simulink model "feedback_lin_EKF"  (R2023b)
settings: Solver=VariableStepAuto  StartTime=0.0  StopTime=2  RelTol=1e-3
values from neighbouring files (symbols this model uses):
  A_ob = A - L*C    [main_feedback_lin.m]
  B_ob = [ B - L*D, L]    [main_feedback_lin.m]
  C_ob = eye(n)    [main_feedback_lin.m]
  D_ob = zeros(n, m+p)    [main_feedback_lin.m]
  m = 1    [main_feedback_lin.m]
undefined symbols (not defined in the file or in its folder): k_aero, k_mag, Lc, Rtot, x1_eq0, x2_eq0, y0
libraries: simulink x3
settings Model: Creator=lollo  LastModifiedBy=lollo

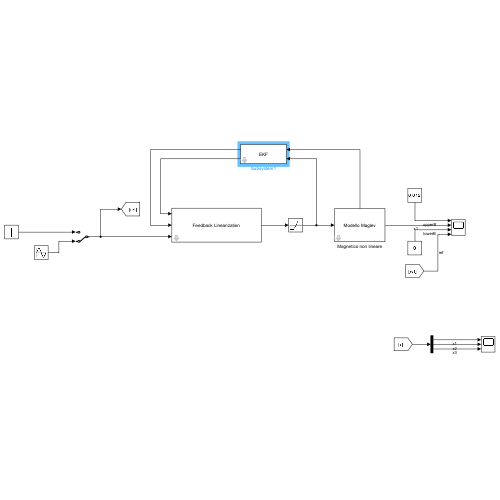
[thumbnail: Simulink's stored preview of the top-level diagram]
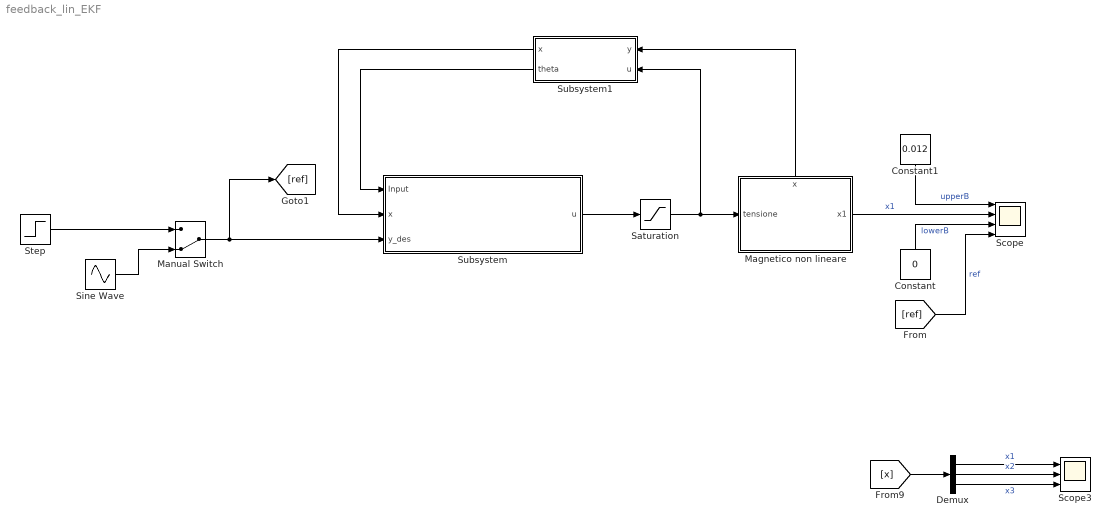
== system feedback_lin_EKF ==
  Constant : Constant  Value=0
  Constant1 : Constant  Value=0.012
  Demux : Demux  Outputs=3
  Magnetico non lineare : Subsystem  mask{dist=on, obs=on, k_aero=k_aero, k_mag=k_mag, m=m, y0=y0, Rtot=Rtot, Lc=Lc}
      mask prompts: dist "Aggiungere Disturbi"; obs "Observer invece di misura"
      settings: PortSchema="{\"entries\":[{\"content\":{\"sides\":[{\"content\":{\"connectorIds\":[\"In1\"]},\"type\":\"ConnectorPlacement.EquallySpacedRectSide\",\"uuid\":\"4c2628b7-19c4-4753-accd-078547eff280\"},{\"content\":{\"connectorIds\":[\"Out1\"],\"side\":\"RIGHT\"},\"type\":\"ConnectorPlacement.EquallySpacedRectSide\",\"uuid\":\"46f8a782-99b4-4db5-ac9e-879226864e1a\"},{\"content\":{\"connectorIds\":[\"Out2\"],\"side\":\"TOP\"},\"type\":\"ConnectorPlacement.EquallySpacedRectSide\",\"uuid\":\"e9ea6a3a-0b10-4f27-be26-5b91ce6de957\"}]},\"type\":\"ConnectorPlacement.EquallySpacedConnector\",\"uuid\":\"8380a659-82e1-48e4-be7e-4b84feeb9f50\"}],\"packageUris\":[\"http://schema.mathworks.com/mf0/Connector/R2020b\"],\"version\":\"1.0\"}"
      mask DialogControl DescGroupVar Prompt: MAGLEV
      mask DialogControl Maglev Prompt: Possibilità di aggiungere disturbi alla misura o di considerare gli observer (solo ridotto alla velocità). Inoltre possibilità di modificare i parametri del modello per testare robustezza
      mask DialogControl Disturbi Prompt: Disturbi
      mask DialogControl Parametri Prompt: Parametri Modello
      mask Display: disp('Modello Maglev')
  Manual Switch : ManualSwitch  CurrentSetting=0
  Saturation : Saturate  UpperLimit=23  LowerLimit=0
  Scope : Scope  NumInputPorts=4
  Scope3 : Scope  NumInputPorts=3
  Sine Wave : Sin  Amplitude=0.001  Bias=0.004  Frequency=10  SampleTime=0
  Step : Step  Time=0  After=0.008  SampleTime=0
  Subsystem : Subsystem  mask{tau=0.003, p1=-100, p2=-60, p3=-70}
      mask DialogControl DescGroupVar Prompt: Feedback Linearization
      mask DialogControl DescTextVar Prompt: Tau corrisponde al tempo caratteristico del filtro per il calcolo delle derivate. k1, k2, k3 sono i poli della feedback linearization dei rispettivi stati
      mask Display: disp('Feedback Linearization')
  Subsystem1 : Subsystem
      mask Display: disp('EKF')
  wires:
  Magnetico non lineare/1(x1) -> Scope/2  "x1"
  Manual Switch/1 -> [ref], Subsystem/3(y_des)
  Subsystem/1(u) -> Saturation/1
  Saturation/1 -> Subsystem1/2(u), Magnetico non lineare/1(tensione)
  Constant/1 -> Scope/3  "lowerB"
  Constant1/1 -> Scope/1  "upperB"
  [x] -> Demux/1
  Demux/2 -> Scope3/2  "x2"
  Demux/3 -> Scope3/3  "x3"
  Demux/1 -> Scope3/1  "x1"
  [ref] -> Scope/4  "ref"
  Step/1 -> Manual Switch/1
  Sine Wave/1 -> Manual Switch/2
  Magnetico non lineare/2(x) -> Subsystem1/1(y)
  Subsystem1/1(x) -> Subsystem/2(x)
  Subsystem1/2(theta) -> Subsystem/1(Input)

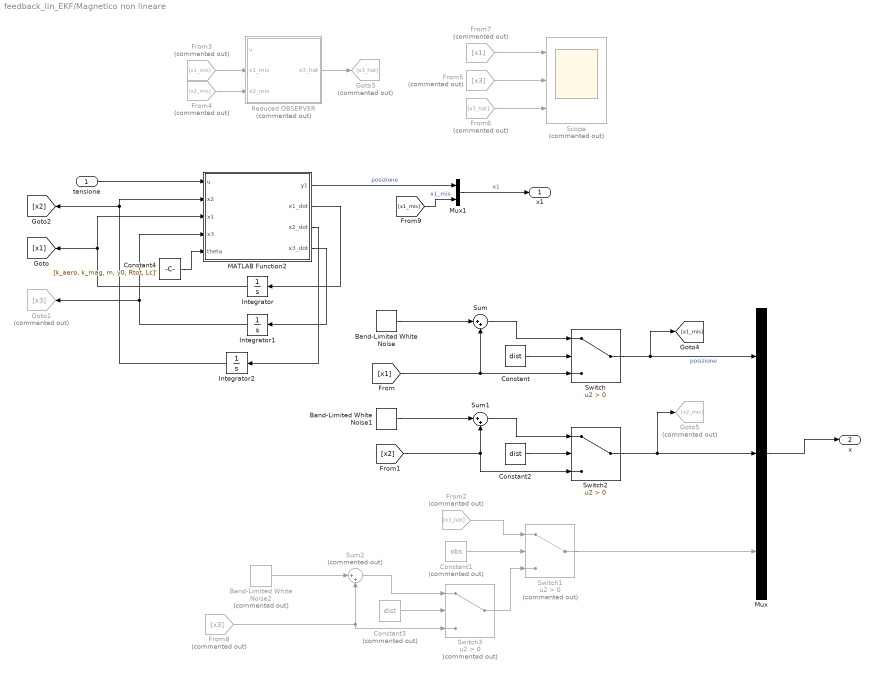
== system feedback_lin_EKF/Magnetico non lineare ==
  tensione : Inport
  Band-Limited White Noise : simulink/Sources/Band-Limited White Noise  Cov=[8.9934e-11*0.002]  Ts=0.002  seed=[23341]
  Band-Limited White Noise1 : simulink/Sources/Band-Limited White Noise  Cov=[8.9934e-11*0.002]  Ts=0.002  seed=[23341]
  Band-Limited White Noise2 : simulink/Sources/Band-Limited White Noise  Commented=on  Cov=[8.9934e-11*0.002]  Ts=0.002  seed=[23341]
  Constant : Constant  Value=dist
  Constant1 : Constant  Commented=on  Value=obs
  Constant2 : Constant  Value=dist
  Constant3 : Constant  Commented=on  Value=dist
  Constant4 : Constant  Value=[k_aero, k_mag, m, y0, Rtot, Lc]'
  From2 : From  Commented=on  GotoTag=x3_hat
  From3 : From  Commented=on  GotoTag=x1_mis
  From4 : From  Commented=on  GotoTag=x2_mis
  From5 : From  Commented=on  GotoTag=x3
  From6 : From  Commented=on  GotoTag=x3_hat
  From7 : From  Commented=on  GotoTag=x1
  From8 : From  Commented=on  GotoTag=x3
  Goto1 : Goto  Commented=on  GotoTag=x3
  Goto3 : Goto  Commented=on  GotoTag=x3_hat
  Goto5 : Goto  Commented=on  GotoTag=x2_mis
  Integrator : Integrator
  Integrator1 : Integrator
  Integrator2 : Integrator
  MATLAB Function2 : MATLAB Function  TreatAsAtomicUnit=on
  Mux : Mux  Inputs=3
  Mux1 : Mux  Inputs=2
  Reduced OBSERVER : Subsystem  Commented=on
  Scope : Scope  Commented=on  NumInputPorts=3
  Sum : Sum  Inputs=|++
  Sum1 : Sum  Inputs=|++
  Sum2 : Sum  Commented=on  Inputs=|++
  Switch : Switch  Criteria=u2 > Threshold  SaturateOnIntegerOverflow=off  InputSameDT=off
  Switch1 : Switch  Commented=on  Criteria=u2 > Threshold  SaturateOnIntegerOverflow=off  InputSameDT=off
  Switch2 : Switch  Criteria=u2 > Threshold  SaturateOnIntegerOverflow=off  InputSameDT=off
  Switch3 : Switch  Commented=on  Criteria=u2 > Threshold  SaturateOnIntegerOverflow=off  InputSameDT=off
  x1 : Outport
  x : Outport  Port=2
  wires:
  tensione/1 -> MATLAB Function2/1(u)
  Switch/1 -> [x1_mis], Mux/1  "posizione"
  MATLAB Function2/2(x1_dot) -> Integrator/1
  Integrator/1 -> MATLAB Function2/3(x1), [x1]
  MATLAB Function2/4(x3_dot) -> Integrator1/1
  Integrator1/1 -> Goto1/1, MATLAB Function2/4(x3)
  [x1] -> Sum/2, Switch/3
  From2/1 -> Switch1/1
  Mux/1 -> x/1
  MATLAB Function2/3(x2_dot) -> Integrator2/1
  From3/1 -> Reduced OBSERVER/2(x1_mis)
  From4/1 -> Reduced OBSERVER/3(x2_mis)
  Reduced OBSERVER/1(x3_hat) -> Goto3/1
  From6/1 -> Scope/3
  From5/1 -> Scope/2
  Integrator2/1 -> [x2], MATLAB Function2/2(x2)
  From7/1 -> Scope/1
  Constant/1 -> Switch/2
  Band-Limited White Noise/1 -> Sum/1
  Sum/1 -> Switch/1
  Constant1/1 -> Switch1/2
  Switch1/1 -> Mux/3
  Constant2/1 -> Switch2/2
  Switch2/1 -> Goto5/1, Mux/2
  Band-Limited White Noise1/1 -> Sum1/1
  Sum1/1 -> Switch2/1
  [x2] -> Sum1/2, Switch2/3
  Constant3/1 -> Switch3/2
  Switch3/1 -> Switch1/3
  Band-Limited White Noise2/1 -> Sum2/1
  Sum2/1 -> Switch3/1
  From8/1 -> Sum2/2, Switch3/3
  [x1_mis] -> Mux1/2  "x1_mis"
  MATLAB Function2/1(y1) -> Mux1/1  "posizione"
  Mux1/1 -> x1/1  "x1"
  Constant4/1 -> MATLAB Function2/5(theta)

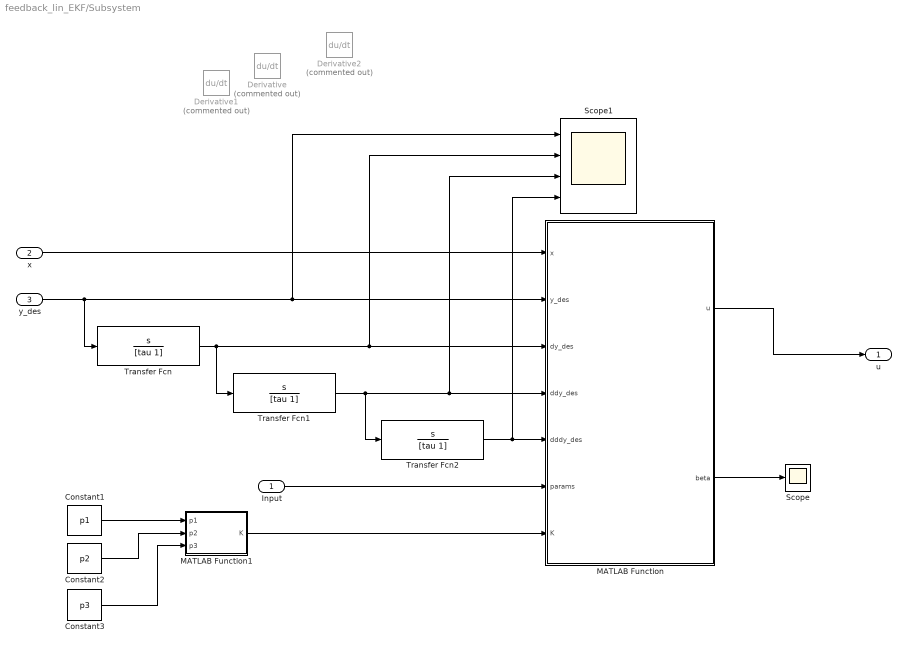
== system feedback_lin_EKF/Subsystem ==
  Input : Inport
  x : Inport  Port=2
  y_des : Inport  Port=3
  Constant1 : Constant  Value=p1
  Constant2 : Constant  Value=p2
  Constant3 : Constant  Value=p3
  Derivative : Derivative  Commented=on
  Derivative1 : Derivative  Commented=on
  Derivative2 : Derivative  Commented=on
  MATLAB Function : MATLAB Function  TreatAsAtomicUnit=on
  MATLAB Function1 : MATLAB Function  TreatAsAtomicUnit=on
  Scope : Scope
  Scope1 : Scope  NumInputPorts=4
  Transfer Fcn : TransferFcn  Numerator=[1 0]  Denominator=[tau 1]
  Transfer Fcn1 : TransferFcn  Numerator=[1 0]  Denominator=[tau 1]
  Transfer Fcn2 : TransferFcn  Numerator=[1 0]  Denominator=[tau 1]
  u : Outport
  wires:
  y_des/1 -> Transfer Fcn/1, MATLAB Function/2(y_des), Scope1/1
  x/1 -> MATLAB Function/1(x)
  MATLAB Function/1(u) -> u/1
  Transfer Fcn/1 -> MATLAB Function/3(dy_des), Scope1/2, Transfer Fcn1/1
  Input/1 -> MATLAB Function/6(params)
  Transfer Fcn1/1 -> Transfer Fcn2/1, Scope1/3, MATLAB Function/4(ddy_des)
  MATLAB Function/2(beta) -> Scope/1
  Transfer Fcn2/1 -> Scope1/4, MATLAB Function/5(dddy_des)
  MATLAB Function1/1(K) -> MATLAB Function/7(K)
  Constant3/1 -> MATLAB Function1/3(p3)
  Constant2/1 -> MATLAB Function1/2(p2)
  Constant1/1 -> MATLAB Function1/1(p1)

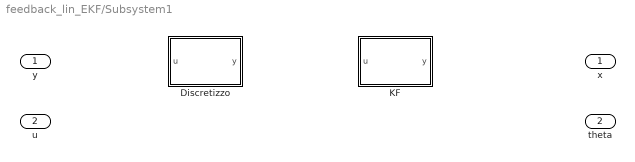
== system feedback_lin_EKF/Subsystem1 ==
  y : Inport
  u : Inport  Port=2
  Discretizzo : MATLAB Function  TreatAsAtomicUnit=on
  KF : MATLAB Function  TreatAsAtomicUnit=on
  x : Outport
  theta : Outport  Port=2

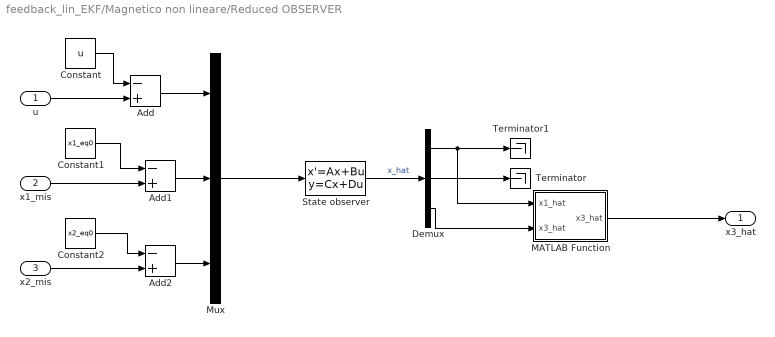
== system feedback_lin_EKF/Magnetico non lineare/Reduced OBSERVER ==
  u : Inport
  x1_mis : Inport  Port=2
  x2_mis : Inport  Port=3
  Add : Sum  Inputs=-+
  Add1 : Sum  Inputs=-+
  Add2 : Sum  Inputs=-+
  Constant : Constant  Value=u
  Constant1 : Constant  Value=x1_eq0
  Constant2 : Constant  Value=x2_eq0
  Demux : Demux  Outputs=3
  MATLAB Function : MATLAB Function  TreatAsAtomicUnit=on
  Mux : Mux  Inputs=3
  State observer : StateSpace  A=A_ob  B=B_ob  C=C_ob  D=D_ob  InitialCondition=[0;0;0]  ParameterTunability=Unconstrained
  Terminator : Terminator
  Terminator1 : Terminator
  x3_hat : Outport
  wires:
  x1_mis/1 -> Add1/2
  u/1 -> Add/2
  Mux/1 -> State observer/1
  State observer/1 -> Demux/1  "x_hat"
  Demux/1 -> MATLAB Function/1(x1_hat), Terminator1/1
  Demux/2 -> Terminator/1
  Constant/1 -> Add/1
  Constant1/1 -> Add1/1
  Constant2/1 -> Add2/1
  x2_mis/1 -> Add2/2
  Add/1 -> Mux/1
  Add1/1 -> Mux/2
  Add2/1 -> Mux/3
  MATLAB Function/1(x3_hat) -> x3_hat/1
  Demux/3 -> MATLAB Function/2("x3_hat ")

== matlab function feedback_lin_EKF/Magnetico non lineare/Reduced OBSERVER/MATLAB Function ==
  data: x1_hat input; x3_hat output; x3_hat input
function x3_hat = fcn(x1_hat, x3_hat)

    if x1_hat<=0 && x3_hat<=0
        x3_hat=0;
    end
end

== matlab function feedback_lin_EKF/Subsystem/MATLAB Function ==
  data: x input; u output; y_des input; dy_des input; ddy_des input; dddy_des input; params input; K input; beta output
function [u, beta] = feedback_linearization_control(x, y_des, dy_des, ddy_des, dddy_des, params, K)
    % Estrai parametri
    k_aero = params(1);
    k_mag  = params(2);
    m      = params(3);
    y0     = params(4);
    Rtot   = params(5);
    Lc     = params(6);
    g      = 9.81;

    % Stati
    x1 = x(1); % posizione
    x2 = x(2); % corrente
    x3 = x(3); % velocità

    % Derivate
    denom = (y0 - x1);
    if denom <= 0
        error('Denominatore nullo o negativo: instabilità elettromagnetica');
    end

    % Accelerazione reale
    xdot3 = (k_aero/m)*x3 + (k_mag/m)*(x2 / denom)^2 - g;

    % Derivate parziali
    dBdx1 = (2 * k_mag * x2^2) / (m * denom^3);
    dBdx2 = (2 * k_mag * x2)   / (m * denom^2);
    dBdx3 = (k_aero/m);

    % Corrente senza ingresso (per calcolo alpha)
    dx2_nou = -(Rtot/Lc)*x2;

    % Parte non lineare (α) e lineare (β)
    alpha = dBdx1 * x3 + dBdx2 * dx2_nou + dBdx3 * xdot3;
    beta  = dBdx2 * (1/Lc);

    if abs(beta) < 1e-6
        warning('Beta troppo piccolo: possibile instabilità numerica');
        u = 5;
        return;
    end

    % Errore e controllore
    e   = x1 - y_des;
    de  = x3 - dy_des;
    ae  = xdot3 - ddy_des;

    

    % Guadagni
    k1 = K(1);
    k2 = K(2);
    k3 = K(3);
    

    % Ingresso virtuale
    % v = p(1, 1)*dddy_des + p(1, 2)*e + p(1, 3)*de + p(1, 4)*ae;
    v = dddy_des - k1*e - k2*de - k3*ae;
    % v = -k1*x1 - k2*x2 - k3*x3;

    % Controllo reale
    u = (v - alpha) / beta;
end

== matlab function feedback_lin_EKF/Subsystem/MATLAB Function1 ==
  data: p1 input; K output; p2 input; p3 input
function K = fcn(p1, p2, p3)

    desired_roots = [p1, p2, p3];
    coeff = poly(desired_roots);     % s^3 + a2*s^2 + a1*s + a0
    K = fliplr(coeff(2:end));

== matlab function feedback_lin_EKF/Magnetico non lineare/MATLAB Function2 ==
  data: u input; y1 output; x2 input; x1_dot output; x2_dot output; x1 input; x3 input; x3_dot output; theta input
function [y1,x1_dot, x2_dot, x3_dot] = fcn(u, x2, x1, x3, theta)
    k_aero = theta(1, 1);
    k_mag = theta(2, 1);
    m = theta(3, 1);
    y0 = theta(4, 1);
    Rtot = theta(5, 1);
    Lc = theta(6, 1);
    g = 9.81;
    
    x2_dot = 1/Lc*(-Rtot*x2 + u);

    x1_dot = x3;
    if x1 < y0
        x3_dot = (k_mag/m)*(x2/(y0-x1))^2 - g;
    else
        x1 = 0.012;
        x3_dot = 0;
        x3 = 0;
    end

    
    % condizioni
    if x1 <=0 && x3_dot < 0
        x1 = 0;
        x3 = 0;
        x3_dot = 0;
    end
y1 = x1;

== matlab function feedback_lin_EKF/Subsystem1/Discretizzo ==
  data: u input; y output
function y = fcn(u)

y = u;

== matlab function feedback_lin_EKF/Subsystem1/KF ==
  data: u input; y output
function y = fcn(u)

y = u;
